simulink model "testrig_susp_linkage_decoupled"  (R2022a)
settings: Solver=ode23t  StartTime=0.0  StopTime=192  MaxStep=0.05  RelTol=1e-3  AbsTol=1e-3  EnableMultiTasking=on
PostLoadFcn:
  | sm_car_load_vehicle_data(bdroot,'206');
  | Vehicle = sm_car_vehcfg_setPeopleOnOff(Vehicle,[0 0 0 0 0],'SuspA1');
  | 
  | Maneuver = sm_car_maneuverdata_knc(0.05,-0.03,0.01,1.25,0.03,500,1200,1200);
  | Visual = sm_car_param_visual('fsae');
undefined symbols (not defined in the file or in its folder): Axle1D, AxleIn, Init, RaceFix, RaceSpin, X, Y, Z
libraries: sm_lib x8, sm_car_testrig_utilities_lib x6, fl_lib x4, Damper_Element x2, Spring_Element x2, nesl_utility x1, Suspension_Linkage_Decoupled x1
CloseFcn:
  | clear simlog_sm_car_testrig_quarter_car
  | clear logsout_sm_car_testrig_quarter_car
Description:
  | Half Car Testrig, Pullrod
  | 
  | Copyright 2021-2024 The MathWorks, Inc.
settings Model: Creator=smiller  LastModifiedBy=smiller
settings SolverCC: AutoScaleAbsTol=off  AlgebraicLoopSolver=TrustRegion
settings DataIOCC: LimitDataPoints=on  MaxDataPoints=10000  ReturnWorkspaceOutputs=off  SignalLoggingName=logsout_sm_car_testrig_quarter_car
settings OptimizationCC: LifeSpan=inf
settings DebuggingCC: UnconnectedInputMsg=warning  UnconnectedOutputMsg=warning  UnconnectedLineMsg=warning  AllowSymbolicDim=off  SFUnexpectedBacktrackingDiag=warning  SFNoUnconditionalDefaultTransitionDiag=warning  SFExecutionAtInitializationDiag=none  SFMachineParentedDataDiag=warning  ArithmeticOperatorsInVariantConditions=warning
settings SFSimCC: SimUseLocalCustomCode=off  CustomCodeUndefinedFunction=UseInterfaceOnly
settings RTWCC: RTWUseLocalCustomCode=off
settings CodeAppCC: StateflowObjectComments=on
settings GRTTargetCC: TargetLangStandard=C89/C90 (ANSI)
settings ConfigComp: CovMetricSettings=dw  CovSaveCumulativeToWorkspaceVar=on  CovSaveSingleToWorkspaceVar=on  CovExternalEMLEnable=off  CovSFcnEnable=off
settings SimscapeCC: SimscapeLogType=all  SimscapeLogSimulationStatistics=on  SimscapeLogName=simlog_sm_car_testrig_quarter_car  SimscapeLogLimitData=off  SimscapeLogDataHistory=10000  SimscapeOperatingPoint=op
settings DiagnosticsConfigSet: SimMechanicsUnconnectedFramePorts=none  SimMechanicsConflictingReferenceFrames=none
settings ExplorerConfigSet: InternalSimMechanicsExplorerSettings="<ExplorerConfiguration><canonicalview>default</canonicalview><AnimationSetting><BasePlaybackSpeed>1.0</BasePlaybackSpeed><PlaybackSpeedFactor>16.0</PlaybackSpeedFactor></AnimationSetting><TilePanel><TileInfo><Tiles Columns=\"1\" Count=\"1\" Rows=\"1\"><Column Weight=\"1\"/><Row Weight=\"1\"/><Tile Height=\"1\" Width=\"1\" X=\"0\" Y=\"0\"/></Tiles></TileInfo><SceneInfo><SceneViewer><BGColor><R>1</R><G>1</G><B>1</B></BGColor><Camera><DoPerspective>off</DoPerspective><Position><X>0.571928528858414942</X><Y>-0.579111562749420217</Y><Z>0.83606068842340453</Z></Position><Center><X>-0.00542174033121090027</X><Y>-0.00176129355979437463</Y><Z>0.258710419233778688</Z></Center><Up><X>-0.408248290463863073</X><Y>0.408248290463863073</Y><Z>0.816496580927726145</Z></Up><ViewLimDist>1</ViewLimDist><YLim>0.718679582981457732</YLim><XLim>0.891323281686500546</XLim></Camera></SceneViewer></SceneInfo></TilePanel><MechEditorPanel><Cameras/><GfxPanelCameraMap/><VideoCreator><PlaybackSpeedRatio>1.0</PlaybackSpeedRatio><FrameRate>30</FrameRate><VideoFormat>Motion JPEG AVI</VideoFormat><FrameSize>auto</FrameSize></VideoCreator></MechEditorPanel></ExplorerConfiguration>"

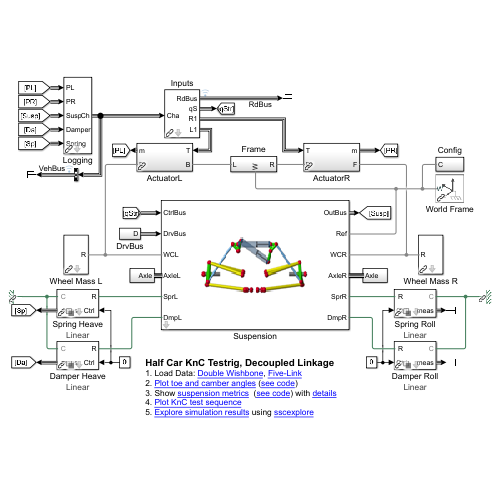
[thumbnail: Simulink's stored preview of the top-level diagram]
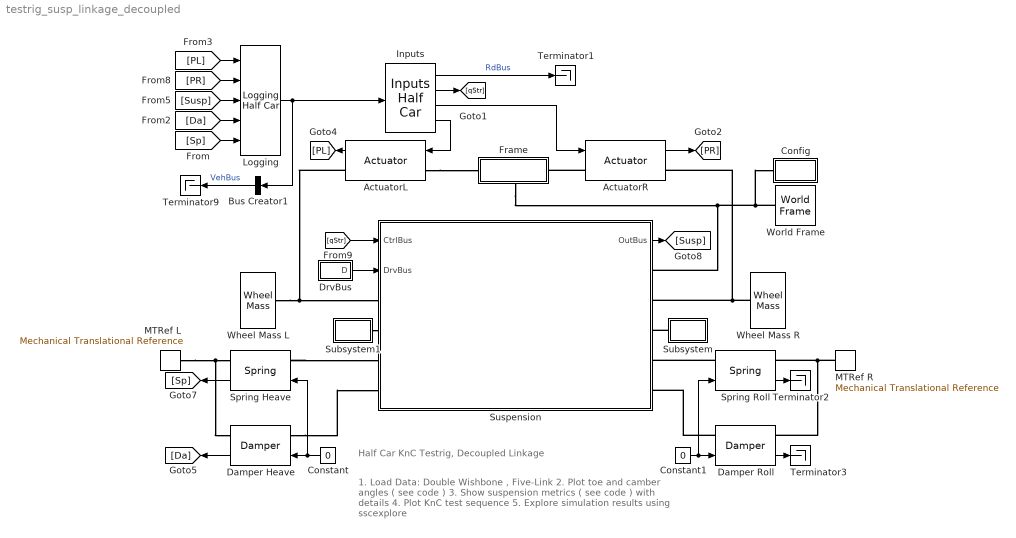
== system testrig_susp_linkage_decoupled ==
  note: Half Car KnC Testrig, Decoupled Linkage
  note: 1. Load Data: Double Wishbone , Five-Link
      | 2. Plot toe and camber angles ( see code )
      | 3. Show suspension metrics ( see code ) with details
      | 4. Plot KnC test sequence
      | 5. Explore simulation results using sscexplore
  ActuatorL : sm_car_testrig_utilities_lib/Actuator  SystemSampleTime=-1  VariantActivationTime=update diagram  Latency=0  AutoFrameSizeCalculation=off
  ActuatorR : sm_car_testrig_utilities_lib/Actuator  SystemSampleTime=-1  VariantActivationTime=update diagram  Latency=0  AutoFrameSizeCalculation=off
  Bus Creator1 : BusCreator  Inputs=1
  Config : Subsystem
  Constant : Constant  Value=0
  Constant1 : Constant  Value=0
  Damper Heave : Damper_Element/Damper  VariantControl=Variant1  LabelModeActiveChoice=Linear  Damper=Vehicle.Chassis.Damper.Axle1.Heave  VariantLabel=Vehicle.Chassis.Damper.Axle1.Heave.class.Value
      settings: AttributesFormatString=%<ActiveVariant>
  Damper Roll : Damper_Element/Damper  VariantControl=Variant1  LabelModeActiveChoice=Linear  Damper=Vehicle.Chassis.Damper.Axle1.Roll  VariantLabel=Vehicle.Chassis.Damper.Axle1.Roll.class.Value
      settings: AttributesFormatString=%<ActiveVariant>
  DrvBus : Subsystem
  Frame : Subsystem
      settings: PortSchema="{\"entries\":[{\"content\":{\"sides\":[{\"content\":{\"connectorIds\":[\"LConn1\"]},\"type\":\"ConnectorPlacement.EquallySpacedRectSide\",\"uuid\":\"4d1860d1-8382-4b55-85c2-09349d56bb16\"},{\"content\":{\"connectorIds\":[\"RConn1\"],\"side\":\"RIGHT\"},\"type\":\"ConnectorPlacement.EquallySpacedRectSide\",\"uuid\":\"4e90683f-4b1a-48f4-aa4c-ab416257a32f\"},{\"content\":{\"connectorIds\":[],\"side\":\"TOP\"},\"type\":\"ConnectorPlacement.EquallySpacedRectSide\",\"uuid\":\"73ac831e-e43d-4cda-a295-19295eab84b4\"},{\"content\":{\"connectorIds\":[\"RConn2\"],\"side\":\"BOTTOM\"},\"type\":\"ConnectorPlacement.EquallySpacedRectSide\",\"uuid\":\"24788d71-0cf9-496d-9e47-2bd8b288be51\"}]},\"type\":\"ConnectorPlacement.EquallySpacedConnector\",\"uuid\":\"859ec081-8f6e-43e9-9a98-d438cbc0fcb8\"}],\"packageUris\":[\"http://schema.mathworks.com/mf0/Connector/R2020b\"],\"version\":\"1.0\"}"
  Inputs : sm_car_testrig_utilities_lib/Inputs Half Car  popup_steering_input=On
  Logging : sm_car_testrig_utilities_lib/Logging Half Car
  MTRef L : fl_lib/Mechanical/Translational Elements/Mechanical Translational Reference
      settings: SourceProductBaseCode=PW,SS,VE
  MTRef R : fl_lib/Mechanical/Translational Elements/Mechanical Translational Reference
      settings: SourceProductBaseCode=PW,SS,VE
  Spring Heave : Spring_Element/Spring  VariantControl=Variant1  LabelModeActiveChoice=Linear  Spring=Vehicle.Chassis.Spring.Axle1.Heave  VariantLabel=Vehicle.Chassis.Spring.Axle1.Heave.class.Value
      settings: AttributesFormatString=%<ActiveVariant>
  Spring Roll : Spring_Element/Spring  VariantControl=Variant1  LabelModeActiveChoice=Linear  Spring=Vehicle.Chassis.Spring.Axle1.Roll  VariantLabel=Vehicle.Chassis.Spring.Axle1.Roll.class.Value
      settings: AttributesFormatString=%<ActiveVariant>
  Subsystem : Subsystem
  Subsystem1 : Subsystem
  Suspension : Subsystem  mask{Susp=Vehicle.Chassis.SuspA1, Init=Init.Axle1}
      mask prompts: Susp "Suspension Parameters (struct)"; Init "Initialization"
      mask Display: image('sm_car_vehicle_susp_linkage_decouple_IMAGE.png');
  Terminator{1..3,9} (4 alike) : Terminator
  Wheel Mass L : sm_car_testrig_utilities_lib/Wheel Mass  tire_param=Vehicle.Chassis.TireA1.tirFile.Value
  Wheel Mass R : sm_car_testrig_utilities_lib/Wheel Mass  tire_param=Vehicle.Chassis.TireA1.tirFile.Value
  World Frame : sm_lib/Frames and Transforms/World Frame
  wires:
  ActuatorR/1 -> [PR]
  Bus Creator1/1 -> Terminator9/1  "VehBus"
  ActuatorL/1 -> [PL]
  Logging/1 -> Inputs/1, Bus Creator1/1
  Inputs/4 -> ActuatorL/1
  Inputs/3 -> ActuatorR/1
  Inputs/2 -> [qStr]
  Inputs/1 -> Terminator1/1  "RdBus"
  [qStr] -> Suspension/1(CtrlBus)
  Suspension/1(OutBus) -> [Susp]
  DrvBus/1(D) -> Suspension/2(DrvBus)
  Spring Heave/1 -> [Sp]
  Damper Heave/1 -> [Da]
  Constant/1 -> Spring Heave/1, Damper Heave/1
  Constant1/1 -> Spring Roll/1, Damper Roll/1
  Spring Roll/1 -> Terminator2/1
  Damper Roll/1 -> Terminator3/1
  [Sp] -> Logging/5
  [Susp] -> Logging/3
  [PL] -> Logging/1
  [PR] -> Logging/2
  [Da] -> Logging/4
  connections:
  ActuatorL/RConn1 -- Wheel Mass L/RConn1 -- Suspension/LConn1
  ActuatorL/LConn1 -- Frame/LConn1
  ActuatorR/LConn1 -- Frame/RConn1
  World Frame/RConn1 -- Frame/RConn2 -- Suspension/RConn1 -- Config/RConn1
  Suspension/RConn2 -- Wheel Mass R/RConn1 -- ActuatorR/RConn1
  Subsystem1/LConn1 -- Suspension/LConn2
  Subsystem/LConn1 -- Suspension/RConn3
  Spring Heave/RConn1 -- Damper Heave/RConn1 -- MTRef L/LConn1
  Damper Heave/LConn1 -- Suspension/LConn4
  Spring Heave/LConn1 -- Suspension/LConn3
  MTRef R/LConn1 -- Spring Roll/RConn1 -- Damper Roll/RConn1
  Spring Roll/LConn1 -- Suspension/RConn4
  Damper Roll/LConn1 -- Suspension/RConn5

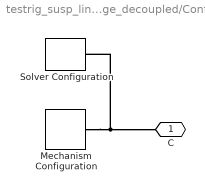
== system testrig_susp_linkage_decoupled/Config ==
  Mechanism Configuration : sm_lib/Utilities/Mechanism Configuration  UniformGravity=Constant  GravityVector=[0 0 -9.80665]  GravityUnits=m/s^2  LinearizationDelta=0.001  JointModeTransitionNonlinearIterations=2
  Solver Configuration : nesl_utility/Solver Configuration  PhysicalDomain=network_engine_domain  SubClassName=solver  LeftPortType=input  RightPortType=generic  Tones=[]  Harmonics=[]  SimulateNoise=off  Profile=off  UseLocalSampling=off  EnableSwitchedLinearOptims=on  FrequencyDomain=off  UseCCode=off  RelTol=0.001  AbsTol=1e-06  MinStep=1e-09  ToWorkspace=off  RevertToSquareIcSolve=off  NumHomotopyIterations=100  PhasorMode=off  PhasorModeNumHarmonics=1  IndexReductionMethod=DerivativeReplacement  DoDC=off  ResidualTolerance=1e-09  UseLocalSolver=off  LocalSolverChoice=NE_BACKWARD_EULER_ADVANCER  LocalSolverSampleTime=0.001  DoFixedCost=off  MaxNonlinIter=3  MaxModeIter=2  ComputeImpulses=off  ImpulseIterations=2  LinearAlgebra=Sparse  LinearAlgebraNumThread=0  EquationFormulation=NE_TIME_EF  DelaysMemoryBudget=1024  AutomaticFiltering=on  FilteringTimeConstant=0.001  PartitionStorageMethod=AS_NEEDED  PartitionMemoryBudget=1024  PartitionMethod=FAST
      settings: SourceProductBaseCode=SS,PW,VE
  C : PMIOPort  Side=Right
  connections:
  Mechanism Configuration/RConn1 -- Solver Configuration/RConn1 -- C/RConn1

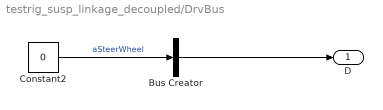
== system testrig_susp_linkage_decoupled/DrvBus ==
  Bus Creator : BusCreator  Inputs=1
  Constant2 : Constant  Value=0
  D : Outport
  wires:
  Constant2/1 -> Bus Creator/1  "aSteerWheel"
  Bus Creator/1 -> D/1

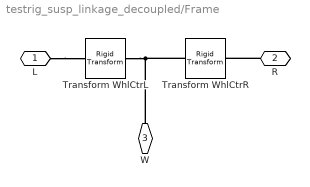
== system testrig_susp_linkage_decoupled/Frame ==
  Transform WhlCtrL : sm_lib/Frames and Transforms/Rigid Transform  TranslationMethod=Cartesian  TranslationStandardOffset=0  TranslationLengthUnit=m  TranslationStandardAxis=+Z  TranslationCartesianOffset=Vehicle.Chassis.SuspA1.Linkage.Upright.sWheelCentre.Value  TranslationROffset=0  TranslationROffsetUnits=m  TranslationZOffset=0  TranslationZOffsetUnits=m  TranslationThetaOffset=0  TranslationThetaOffsetUnits=deg  RotationMethod=None  RotationAngleUnits=deg  RotationStandardAxis=+Z  RotationAngle=0.0  RotationArbitraryAxis=[0 0 1]  FollAlignAxisA=+X  BaseAlignAxisA=+Y  FollAlignAxisB=+Y  BaseAlignAxisB=+Z  RotationSequenceAxes=FollowerAxes  RotationSequence=XYX  RotationSequenceAngles=[0 0 0]  RotationSequenceAnglesUnits=deg  RotationMatrix=[1 0 0; 0 1 0; 0 0 1]
  Transform WhlCtrR : sm_lib/Frames and Transforms/Rigid Transform  TranslationMethod=Cartesian  TranslationStandardOffset=0  TranslationLengthUnit=m  TranslationStandardAxis=+Z  TranslationCartesianOffset=Vehicle.Chassis.SuspA1.Linkage.Upright.sWheelCentre.Value.*[1 -1 1]  TranslationROffset=0  TranslationROffsetUnits=m  TranslationZOffset=0  TranslationZOffsetUnits=m  TranslationThetaOffset=0  TranslationThetaOffsetUnits=deg  RotationMethod=None  RotationAngleUnits=deg  RotationStandardAxis=+Z  RotationAngle=0.0  RotationArbitraryAxis=[0 0 1]  FollAlignAxisA=+X  BaseAlignAxisA=+Y  FollAlignAxisB=+Y  BaseAlignAxisB=+Z  RotationSequenceAxes=FollowerAxes  RotationSequence=XYX  RotationSequenceAngles=[0 0 0]  RotationSequenceAnglesUnits=deg  RotationMatrix=[1 0 0; 0 1 0; 0 0 1]
  L : PMIOPort  Side=Left
  R : PMIOPort  Port=2  Side=Right
  W : PMIOPort  Port=3  Side=Right
  connections:
  R/RConn1 -- Transform WhlCtrR/RConn1
  L/RConn1 -- Transform WhlCtrL/RConn1
  W/RConn1 -- Transform WhlCtrL/LConn1 -- Transform WhlCtrR/LConn1

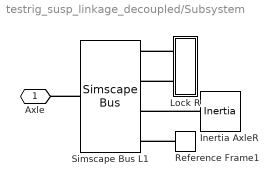
== system testrig_susp_linkage_decoupled/Subsystem ==
  Inertia AxleR : fl_lib/Mechanical/Rotational Elements/Inertia  inertia=0.01 kg*m^2  num_ports=foundation.enum.numPorts2.one  w_specify=on  w_priority=None  w=0 rad/s  w_nominal_specify=off  w_nominal_unit=rad/s  w_nominal_value=1  t_specify=off  t_priority=None  t=0 N*m  t_nominal_specify=off  t_nominal_unit=N*m  t_nominal_value=1
      settings: SourceProductBaseCode=PW,SS,VE
  Lock R : Subsystem
  Reference Frame1 : sm_lib/Frames and Transforms/Reference Frame
  Simscape Bus L1 : SimscapeBus  HierarchyStrings=RaceSpin;RaceFix;Axle1D;AxleIn
  Axle : PMIOPort  Side=Left
  connections:
  Lock R/LConn2 -- Simscape Bus L1/LConn2
  Reference Frame1/RConn1 -- Simscape Bus L1/LConn4
  Lock R/LConn1 -- Simscape Bus L1/LConn1
  Inertia AxleR/LConn1 -- Simscape Bus L1/LConn3
  Simscape Bus L1/RConn1 -- Axle/RConn1

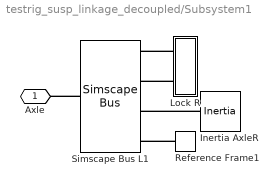
== system testrig_susp_linkage_decoupled/Subsystem1 ==
  Inertia AxleR : fl_lib/Mechanical/Rotational Elements/Inertia  inertia=0.01 kg*m^2  num_ports=foundation.enum.numPorts2.one  w_specify=on  w_priority=None  w=0 rad/s  w_nominal_specify=off  w_nominal_unit=rad/s  w_nominal_value=1  t_specify=off  t_priority=None  t=0 N*m  t_nominal_specify=off  t_nominal_unit=N*m  t_nominal_value=1
      settings: SourceProductBaseCode=PW,SS,VE
  Lock R : Subsystem
  Reference Frame1 : sm_lib/Frames and Transforms/Reference Frame
  Simscape Bus L1 : SimscapeBus  HierarchyStrings=RaceSpin;RaceFix;Axle1D;AxleIn
  Axle : PMIOPort  Side=Left
  connections:
  Simscape Bus L1/RConn1 -- Axle/RConn1
  Inertia AxleR/LConn1 -- Simscape Bus L1/LConn3
  Lock R/LConn1 -- Simscape Bus L1/LConn1
  Reference Frame1/RConn1 -- Simscape Bus L1/LConn4
  Lock R/LConn2 -- Simscape Bus L1/LConn2

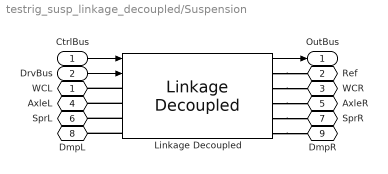
== system testrig_susp_linkage_decoupled/Suspension ==
  CtrlBus : Inport
  DrvBus : Inport  Port=2
  Linkage Decoupled : Suspension_Linkage_Decoupled/Linkage Decoupled  VariantControl=Decoupled
  WCL : PMIOPort  Side=Left
  Ref : PMIOPort  Port=2  Side=Right
  WCR : PMIOPort  Port=3  Side=Right
  AxleL : PMIOPort  Port=4  Side=Left
  AxleR : PMIOPort  Port=5  Side=Right
  SprL : PMIOPort  Port=6  Side=Left
  SprR : PMIOPort  Port=7  Side=Right
  DmpL : PMIOPort  Port=8  Side=Left
  DmpR : PMIOPort  Port=9  Side=Right
  OutBus : Outport
  wires:
  CtrlBus/1 -> Linkage Decoupled/1
  Linkage Decoupled/1 -> OutBus/1
  DrvBus/1 -> Linkage Decoupled/2
  connections:
  Linkage Decoupled/RConn5 -- DmpR/RConn1
  Linkage Decoupled/LConn3 -- SprL/RConn1
  Linkage Decoupled/LConn4 -- DmpL/RConn1
  Linkage Decoupled/RConn2 -- WCR/RConn1
  Linkage Decoupled/RConn4 -- SprR/RConn1
  Linkage Decoupled/RConn3 -- AxleR/RConn1
  Linkage Decoupled/LConn2 -- AxleL/RConn1
  Linkage Decoupled/LConn1 -- WCL/RConn1
  Linkage Decoupled/RConn1 -- Ref/RConn1

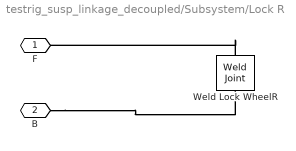
== system testrig_susp_linkage_decoupled/Subsystem/Lock R ==
  Weld Lock WheelR : sm_lib/Joints/Weld Joint  JointMode=Normal  SenseConstraintForce=off  SenseConstraintForceX=off  SenseConstraintForceY=off  SenseConstraintForceZ=off  SenseConstraintTorque=off  SenseConstraintTorqueX=off  SenseConstraintTorqueY=off  SenseConstraintTorqueZ=off  SenseTotalForce=off  SenseTotalForceX=off  SenseTotalForceY=off  SenseTotalForceZ=off  SenseTotalTorque=off  SenseTotalTorqueX=off  SenseTotalTorqueY=off  SenseTotalTorqueZ=off  CompositeWrenchDir=FollowerOnBase  CompositeWrenchFrame=BaseFrame
  F : PMIOPort  Side=Left
  B : PMIOPort  Port=2  Side=Left
  connections:
  Weld Lock WheelR/RConn1 -- F/RConn1
  B/RConn1 -- Weld Lock WheelR/LConn1

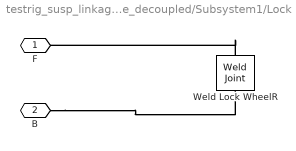
== system testrig_susp_linkage_decoupled/Subsystem1/Lock R ==
  Weld Lock WheelR : sm_lib/Joints/Weld Joint  JointMode=Normal  SenseConstraintForce=off  SenseConstraintForceX=off  SenseConstraintForceY=off  SenseConstraintForceZ=off  SenseConstraintTorque=off  SenseConstraintTorqueX=off  SenseConstraintTorqueY=off  SenseConstraintTorqueZ=off  SenseTotalForce=off  SenseTotalForceX=off  SenseTotalForceY=off  SenseTotalForceZ=off  SenseTotalTorque=off  SenseTotalTorqueX=off  SenseTotalTorqueY=off  SenseTotalTorqueZ=off  CompositeWrenchDir=FollowerOnBase  CompositeWrenchFrame=BaseFrame
  F : PMIOPort  Side=Left
  B : PMIOPort  Port=2  Side=Left
  connections:
  B/RConn1 -- Weld Lock WheelR/LConn1
  Weld Lock WheelR/RConn1 -- F/RConn1
